simulink model "SIMULINK_SYS"  (R2015a)
settings: Solver=ode45  StartTime=0.0  StopTime=15  RelTol=1e-3
libraries: slident x2, simulink x1
settings Model: Creator=Alim Satria  LastModifiedBy=Alim Satria

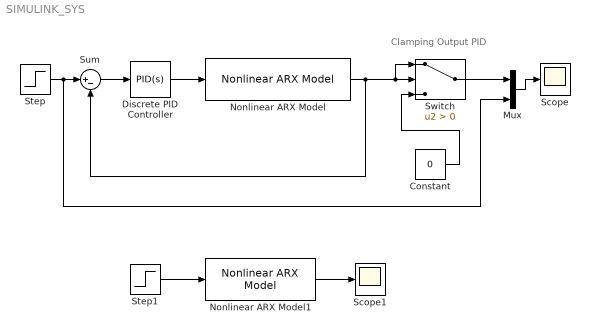
== system SIMULINK_SYS ==
  note: Clamping Output PID
  Constant : Constant  Value=0
  Discrete PID Controller : simulink/Continuous/PID Controller  Controller=PID  TimeDomain=Continuous-time  SampleTime=-1  IntegratorMethod=Forward Euler  FilterMethod=Forward Euler  Form=Parallel  UseFilter=on  ControllerParametersSource=internal  P=1.41353356021094  I=2.64031091824156  D=0.0853909052978635  N=22.9449229808967  InitialConditionSource=internal  InitialConditionForIntegrator=0  InitialConditionForFilter=0  ExternalReset=none  LimitOutput=on  UpperSaturationLimit=1410  LowerSaturationLimit=900  LinearizeAsGain=off  AntiWindupMode=none  Kb=1  TrackingMode=off  Kt=1  PParamMin=[]  PParamMax=[]  IParamMin=[]  IParamMax=[]  DParamMin=[]  DParamMax=[]  NParamMin=[]  NParamMax=[]  KbParamMin=[]  KbParamMax=[]  KtParamMin=[]  KtParamMax=[]  POutMin=[]  POutMax=[]  IOutMin=[]  IOutMax=[]  DOutMin=[]  DOutMax=[]  NOutMin=[]  NOutMax=[]  KbOutMin=[]  KbOutMax=[]  KtOutMin=[]  KtOutMax=[]  IntegratorOutMin=[]  IntegratorOutMax=[]  FilterOutMin=[]  FilterOutMax=[]  SumOutMin=[]  SumOutMax=[]  SumI1OutMin=[]  SumI1OutMax=[]  SumI2OutMin=[]  SumI2OutMax=[]  SumI3OutMin=[]  SumI3OutMax=[]  SumDOutMin=[]  SumDOutMax=[]  SaturationOutMin=[]  SaturationOutMax=[]  IntegratorContinuousStateAttributes=''  IntegratorStateMustResolveToSignalObject=off  IntegratorRTWStateStorageClass=Auto  FilterContinuousStateAttributes=''  FilterStateMustResolveToSignalObject=off  FilterRTWStateStorageClass=Auto  DifferentiatorICPrevScaledInput=0  DifferentiatorOutMin=[]  DifferentiatorOutMax=[]
  Mux : Mux  Inputs=2
  Nonlinear ARX Model : slident/Models/Nonlinear ARX Model  sys=NLARX_DATASET_1_REV  ICspec=Input and output values  X0=0  U0=0  Y0=0
  Nonlinear ARX Model1 : slident/Models/Nonlinear ARX Model  sys=NLARX_DATASET_1_REV  ICspec=Input and output values  X0=0  U0=0  Y0=0
  Scope : Scope
  Scope1 : Scope
  Step : Step  After=350  SampleTime=0.05
  Step1 : Step  After=350  SampleTime=0.05
  Sum : Sum  Inputs=|+-
  Switch : Switch  Criteria=u2 > Threshold
  wires:
  Step/1 -> Mux/2, Sum/1
  Mux/1 -> Scope/1
  Discrete PID Controller/1 -> Nonlinear ARX Model/1
  Sum/1 -> Discrete PID Controller/1
  Nonlinear ARX Model/1 -> Switch/2, Switch/1, Sum/2
  Switch/1 -> Mux/1
  Constant/1 -> Switch/3
  Step1/1 -> Nonlinear ARX Model1/1
  Nonlinear ARX Model1/1 -> Scope1/1
